simulink model "intro"  (R2024b)
settings: Solver=VariableStepAuto  StartTime=0.0  StopTime=100.0  RelTol=1e-3
settings Model: Creator=obe  LastModifiedBy=obe

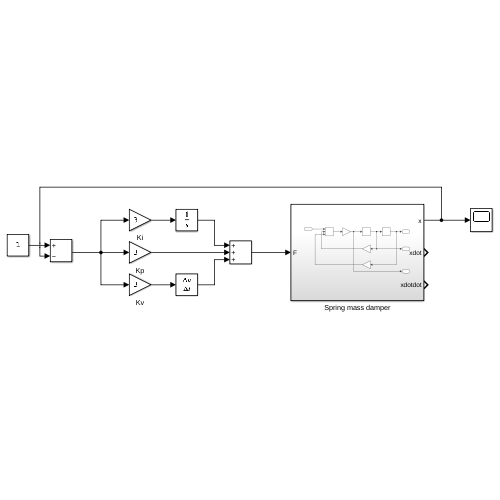
[thumbnail: Simulink's stored preview of the top-level diagram]
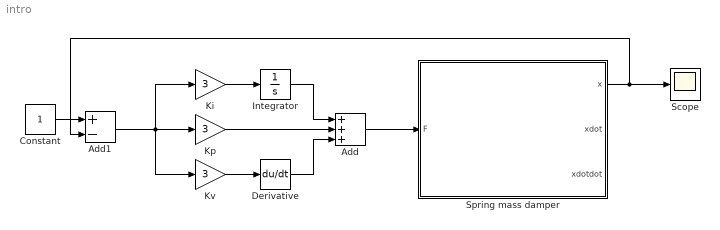
== system intro ==
  Add : Sum  Inputs=+++
  Add1 : Sum  Inputs=+-
  Constant : Constant
  Derivative : Derivative
  Integrator : Integrator
  Ki : Gain  Gain=3
  Kp : Gain  Gain=3
  Kv : Gain  Gain=3
  Scope : Scope
  Spring mass damper : Subsystem
  wires:
  Add/1 -> Spring mass damper/1(F)
  Integrator/1 -> Add/1
  Derivative/1 -> Add/3
  Kp/1 -> Add/2
  Ki/1 -> Integrator/1
  Kv/1 -> Derivative/1
  Add1/1 -> Kv/1, Kp/1, Ki/1
  Spring mass damper/1(x) -> Scope/1, Add1/2
  Constant/1 -> Add1/1

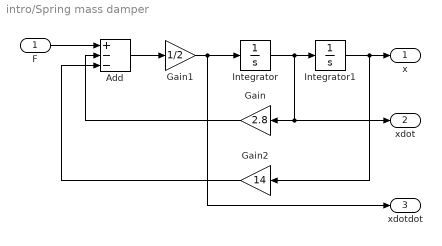
== system intro/Spring mass damper ==
  F : Inport
  Add : Sum  Inputs=+--
  Gain : Gain  Gain=2.8
  Gain1 : Gain  Gain=1/2
  Gain2 : Gain  Gain=14
  Integrator : Integrator
  Integrator1 : Integrator
  x : Outport
  xdot : Outport  Port=2
  xdotdot : Outport  Port=3
  wires:
  Gain2/1 -> Add/3
  Gain/1 -> Add/2
  Integrator1/1 -> x/1, Gain2/1
  F/1 -> Add/1
  Gain1/1 -> xdotdot/1, Integrator/1
  Add/1 -> Gain1/1
  Integrator/1 -> Integrator1/1, xdot/1, Gain/1
